simulink model "electroMagnetModel"  (R2020a)
settings: Solver=ode45  StartTime=0.0  StopTime=5  MaxStep=0.01  RelTol=1e-3  EnableMultiTasking=on
undefined symbols (not defined in the file): k1, k2, k3, Ki, Ks, L, m1, m2, m3, R, u_0, x_0
settings Model: Creator=dimpa  LastModifiedBy=tanzc
settings DataIOCC: LimitDataPoints=on  SaveFormat=Array  ReturnWorkspaceOutputs=off
settings OptimizationCC: LifeSpan=inf
settings DebuggingCC: SolverPrmCheckMsg=warning  SFUnexpectedBacktrackingDiag=warning  SFNoUnconditionalDefaultTransitionDiag=warning  SFExecutionAtInitializationDiag=none  ArithmeticOperatorsInVariantConditions=warning
settings HardwareCC: ProdBitPerPointer=32  ProdBitPerSizeT=32  ProdBitPerPtrDiffT=32  ProdLargestAtomicFloat=None  ProdIntDivRoundTo=Undefined  ProdEndianess=Unspecified  ProdWordSize=32  ProdHWDeviceType=32-bit Generic
settings ModelReferenceCC: PropagateSignalLabelsOutOfModel=off
settings SFSimCC: SimUseLocalCustomCode=off  CustomCodeUndefinedFunction=UseInterfaceOnly
settings RTWCC: RTWUseLocalCustomCode=off
settings CodeAppCC: StateflowObjectComments=on
settings GRTTargetCC: TargetLangStandard=C89/C90 (ANSI)
settings ConfigComp: CovMetricSettings=dw  CovHtmlReporting=on  CovSaveCumulativeToWorkspaceVar=on  CovSaveSingleToWorkspaceVar=on  CovExternalEMLEnable=off  CovSFcnEnable=off

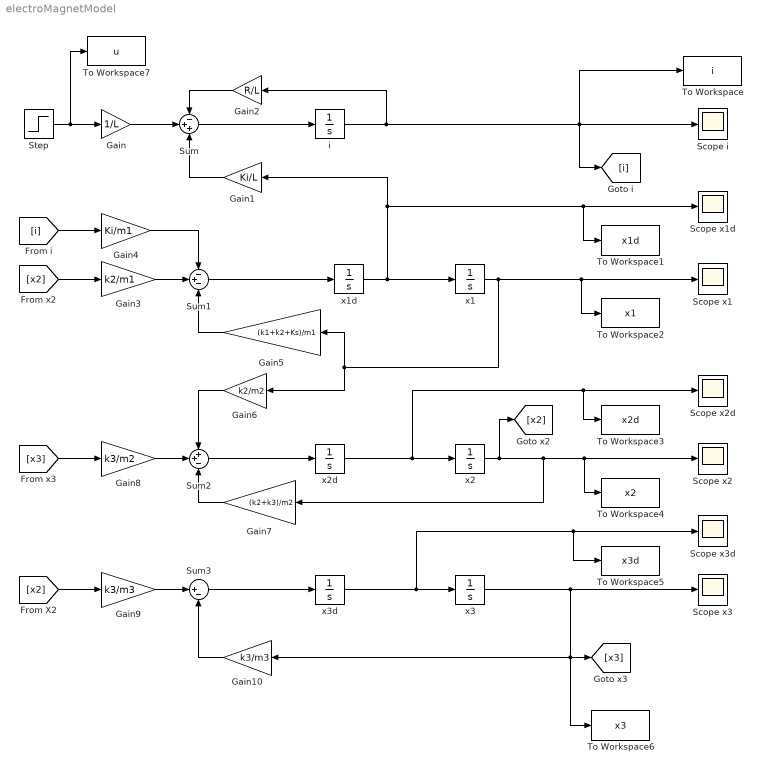
== system electroMagnetModel ==
  Gain : Gain  Gain=1/L
  Gain1 : Gain  Gain=Ki/L
  Gain10 : Gain  Gain=k3/m3
  Gain2 : Gain  Gain=R/L
  Gain3 : Gain  Gain=k2/m1
  Gain4 : Gain  Gain=Ki/m1
  Gain5 : Gain  Gain=(k1+k2+Ks)/m1
  Gain6 : Gain  Gain=k2/m2
  Gain7 : Gain  Gain=(k2+k3)/m2
  Gain8 : Gain  Gain=k3/m2
  Gain9 : Gain  Gain=k3/m3
  Scope i : Scope
  Scope x1 : Scope
  Scope x1d : Scope
  Scope x2 : Scope
  Scope x2d : Scope
  Scope x3 : Scope
  Scope x3d : Scope
  Step : Step  After=u_0  SampleTime=0
  Sum : Sum  Inputs=-++
  Sum1 : Sum  Inputs=-+-
  Sum2 : Sum  Inputs=++-
  Sum3 : Sum  Inputs=|+-
  To Workspace : ToWorkspace  VariableName=i  SaveFormat=Structure With Time  SampleTime=-1
  To Workspace1 : ToWorkspace  VariableName=x1d  SaveFormat=Structure With Time  SampleTime=-1
  To Workspace2 : ToWorkspace  VariableName=x1  SaveFormat=Structure With Time  SampleTime=-1
  To Workspace3 : ToWorkspace  VariableName=x2d  SaveFormat=Structure With Time  SampleTime=-1
  To Workspace4 : ToWorkspace  VariableName=x2  SaveFormat=Structure With Time  SampleTime=-1
  To Workspace5 : ToWorkspace  VariableName=x3d  SaveFormat=Structure With Time  SampleTime=-1
  To Workspace6 : ToWorkspace  VariableName=x3  SaveFormat=Structure With Time  SampleTime=-1
  To Workspace7 : ToWorkspace  VariableName=u  SaveFormat=Structure With Time  SampleTime=-1
  i : Integrator  InitialCondition=x_0(1)
  x1 : Integrator  InitialCondition=x_0(2)
  x1d : Integrator  InitialCondition=x_0(3)
  x2 : Integrator  InitialCondition=x_0(4)
  x2d : Integrator  InitialCondition=x_0(5)
  x3 : Integrator  InitialCondition=x_0(6)
  x3d : Integrator  InitialCondition=x_0(7)
  wires:
  x1d/1 -> To Workspace1/1, Scope x1d/1, Gain1/1, x1/1
  Step/1 -> To Workspace7/1, Gain/1
  Sum/1 -> i/1
  i/1 -> Gain2/1, To Workspace/1, [i], Scope i/1
  Gain2/1 -> Sum/1
  Gain/1 -> Sum/2
  Gain1/1 -> Sum/3
  x1/1 -> Gain5/1, Gain6/1, To Workspace2/1, Scope x1/1
  Gain4/1 -> Sum1/1
  x2/1 -> [x2], Gain7/1, To Workspace4/1, Scope x2/1
  x2d/1 -> To Workspace3/1, Scope x2d/1, x2/1
  x3d/1 -> To Workspace5/1, Scope x3d/1, x3/1
  x3/1 -> To Workspace6/1, [x3], Gain10/1, Scope x3/1
  [i] -> Gain4/1
  [x2] -> Gain3/1
  Gain3/1 -> Sum1/2
  Gain5/1 -> Sum1/3
  Sum1/1 -> x1d/1
  Gain6/1 -> Sum2/1
  [x3] -> Gain8/1
  Gain8/1 -> Sum2/2
  Gain7/1 -> Sum2/3
  Sum2/1 -> x2d/1
  [x2] -> Gain9/1
  Gain9/1 -> Sum3/1
  Gain10/1 -> Sum3/2
  Sum3/1 -> x3d/1
